simulink model "Filter"  (R2020b)
settings: Solver=FixedStepDiscrete  StartTime=0.0  StopTime=100.0  FixedStep=1  RelTol=1e-3
settings Model: Creator=ncleju  LastModifiedBy=ncleju

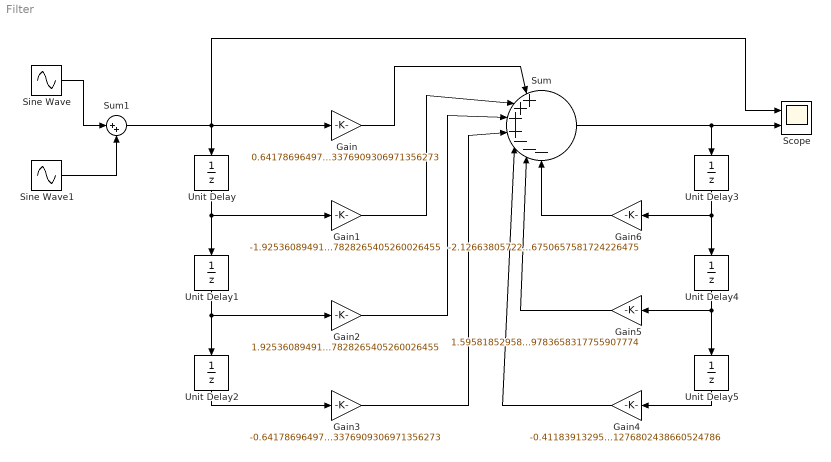
== system Filter ==
  Gain : Gain  Gain=0.641786964970792683793376909306971356273
  Gain1 : Gain  Gain=-1.925360894912377940357828265405260026455
  Gain2 : Gain  Gain=1.925360894912377940357828265405260026455
  Gain3 : Gain  Gain=-0.641786964970792683793376909306971356273
  Gain4 : Gain  Gain=-0.411839132950082509321276802438660524786
  Gain5 : Gain  Gain=1.59581852958974890199783658317755907774
  Gain6 : Gain  Gain=-2.126638057226510003516750657581724226475
  Scope : Scope  NumInputPorts=2
  Sine Wave : Sin  Frequency=2*pi*0.03  Phase=pi/2  SampleTime=0
  Sine Wave1 : Sin  Frequency=2*pi*0.18  Phase=pi/2  SampleTime=0
  Sum : Sum  Inputs=|++++---
  Sum1 : Sum  Inputs=|++
  Unit Delay{,1..5} (6 alike) : UnitDelay  SampleTime=-1  HasFrameUpgradeWarning=on
  wires:
  Gain/1 -> Sum/1
  Unit Delay/1 -> Unit Delay1/1, Gain1/1
  Gain1/1 -> Sum/2
  Unit Delay1/1 -> Unit Delay2/1, Gain2/1
  Gain2/1 -> Sum/3
  Unit Delay2/1 -> Gain3/1
  Gain3/1 -> Sum/4
  Sum/1 -> Unit Delay3/1, Scope/2
  Unit Delay3/1 -> Unit Delay4/1, Gain6/1
  Unit Delay4/1 -> Gain5/1, Unit Delay5/1
  Unit Delay5/1 -> Gain4/1
  Gain6/1 -> Sum/7
  Gain5/1 -> Sum/6
  Gain4/1 -> Sum/5
  Sine Wave/1 -> Sum1/1
  Sine Wave1/1 -> Sum1/2
  Sum1/1 -> Scope/1, Unit Delay/1, Gain/1
